simulink model "Earth_sim"  (R2024b)
settings: Solver=VariableStepAuto  StartTime=0.0  StopTime=15e4  FixedStep=0.5  MaxStep=10  RelTol=1e-6
undefined symbols (not defined in the file): earth_escape_data, Earth_planet, launch_data, launch_site, transfer_outbound_data
settings Model: Creator=cpero  LastModifiedBy=cpero
settings SolverCC: MaxConsecutiveMinStep=10  MinimalZcImpactIntegration=on  EnableFixedStepZeroCrossing=on
settings DebuggingCC: ReadBeforeWriteMsg=DisableAll  WriteAfterWriteMsg=DisableAll  WriteAfterReadMsg=DisableAll  MultiTaskDSMMsg=none
settings ModelReferenceCC: UpdateModelReferenceTargets=IfOutOfDate
settings SFSimCC: SFSimEcho=off

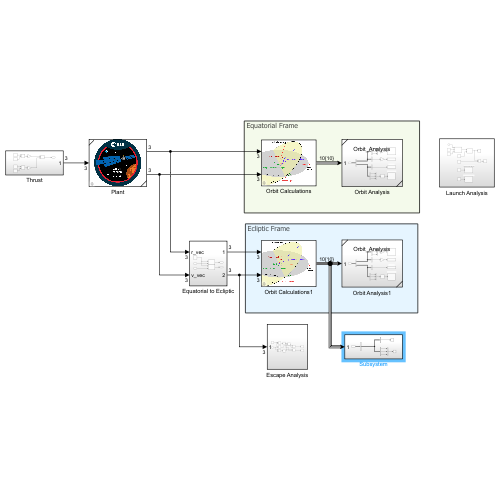
[thumbnail: Simulink's stored preview of the top-level diagram]
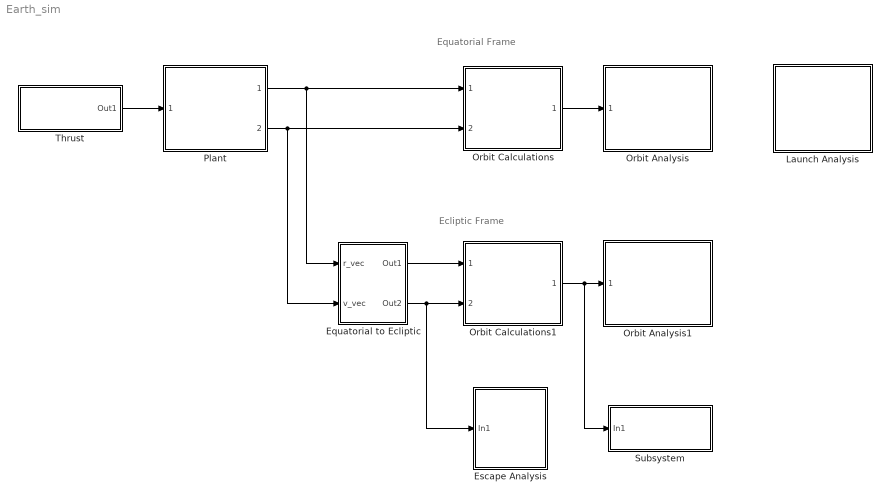
== system Earth_sim ==
  note: Equatorial Frame
  note: Ecliptic Frame
  Equatorial to Ecliptic : Subsystem
  Escape Analysis : Subsystem
  Launch Analysis : Subsystem
  Orbit Analysis : Subsystem  ReferencedSubsystem=Orbit_Analysis
  Orbit Analysis1 : Subsystem  ReferencedSubsystem=Orbit_Analysis
  Orbit Calculations : Subsystem  ReferencedSubsystem=Orbit_Calculations  mu=Earth_planet.mu
  Orbit Calculations1 : Subsystem  ReferencedSubsystem=Orbit_Calculations  mu=Earth_planet.mu
  Plant : Subsystem  ReferencedSubsystem=Plant  setup=launch_data  switch_time=launch_data.wait_time  mu=Earth_planet.mu
  Subsystem : Subsystem
  Thrust : Subsystem
  wires:
  Orbit Calculations/1 -> Orbit Analysis/1
  Plant/1 -> Orbit Calculations/1, Equatorial to Ecliptic/1(r_vec)
  Plant/2 -> Orbit Calculations/2, Equatorial to Ecliptic/2(v_vec)
  Orbit Calculations1/1 -> Subsystem/1(In1), Orbit Analysis1/1
  Equatorial to Ecliptic/1(Out1) -> Orbit Calculations1/1
  Equatorial to Ecliptic/2(Out2) -> Escape Analysis/1(In1), Orbit Calculations1/2
  Thrust/1(Out1) -> Plant/1

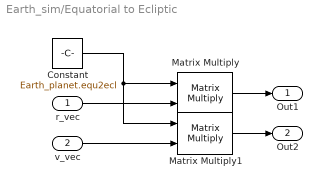
== system Earth_sim/Equatorial to Ecliptic ==
  r_vec : Inport
  v_vec : Inport  Port=2
  Constant : Constant  Value=Earth_planet.equ2ecl
  Matrix Multiply : Product  Multiplication=Matrix(*)
  Matrix Multiply1 : Product  Multiplication=Matrix(*)
  Out1 : Outport
  Out2 : Outport  Port=2
  wires:
  Constant/1 -> Matrix Multiply1/1, Matrix Multiply/1
  Matrix Multiply1/1 -> Out2/1
  Matrix Multiply/1 -> Out1/1
  r_vec/1 -> Matrix Multiply/2
  v_vec/1 -> Matrix Multiply1/2

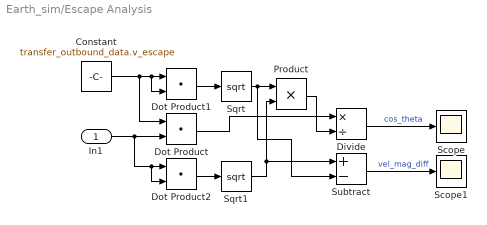
== system Earth_sim/Escape Analysis ==
  In1 : Inport
  Constant : Constant  Value=transfer_outbound_data.v_escape
  Divide : Product  Inputs=*/
  Dot Product : DotProduct  OutDataTypeStr=Inherit: Inherit via internal rule
  Dot Product1 : DotProduct  OutDataTypeStr=Inherit: Inherit via internal rule
  Dot Product2 : DotProduct  OutDataTypeStr=Inherit: Inherit via internal rule
  Product : Product
  Scope : Scope
  Scope1 : Scope
  Sqrt : Sqrt
  Sqrt1 : Sqrt
  Subtract : Sum  Inputs=+-
  wires:
  Constant/1 -> Dot Product1/2, Dot Product1/1, Dot Product/1
  Dot Product1/1 -> Sqrt/1
  Dot Product2/1 -> Sqrt1/1
  In1/1 -> Dot Product2/2, Dot Product2/1, Dot Product/2
  Sqrt/1 -> Subtract/2, Product/1
  Sqrt1/1 -> Product/2, Subtract/1
  Divide/1 -> Scope/1  "cos_theta"
  Product/1 -> Divide/2
  Dot Product/1 -> Divide/1
  Subtract/1 -> Scope1/1  "vel_mag_diff"

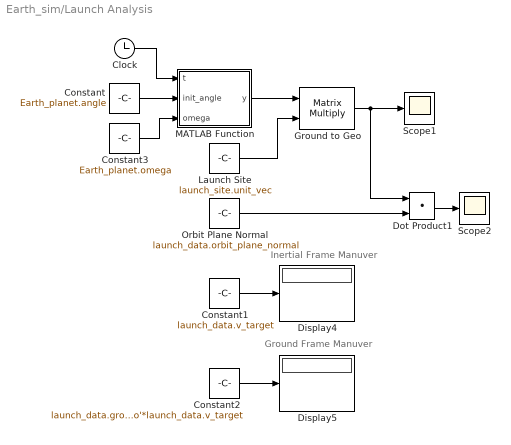
== system Earth_sim/Launch Analysis ==
  note: Ground Frame Manuver
  note: Inertial Frame Manuver
  Clock : Clock
  Constant : Constant  Value=Earth_planet.angle
  Constant1 : Constant  Value=launch_data.v_target
  Constant2 : Constant  Value=launch_data.ground2geo'*launch_data.v_target
  Constant3 : Constant  Value=Earth_planet.omega
  Display4 : Display
  Display5 : Display
  Dot Product1 : DotProduct  OutDataTypeStr=Inherit: Inherit via internal rule
  Ground to Geo : Product  Multiplication=Matrix(*)
  Launch Site : Constant  Value=launch_site.unit_vec
  MATLAB Function : MATLAB Function  TreatAsAtomicUnit=on
  Orbit Plane Normal : Constant  Value=launch_data.orbit_plane_normal
  Scope1 : Scope
  Scope2 : Scope
  wires:
  Dot Product1/1 -> Scope2/1
  Orbit Plane Normal/1 -> Dot Product1/2
  Ground to Geo/1 -> Scope1/1, Dot Product1/1
  Clock/1 -> MATLAB Function/1(t)
  MATLAB Function/1(y) -> Ground to Geo/1
  Launch Site/1 -> Ground to Geo/2
  Constant2/1 -> Display5/1
  Constant1/1 -> Display4/1
  Constant/1 -> MATLAB Function/2(init_angle)
  Constant3/1 -> MATLAB Function/3(omega)

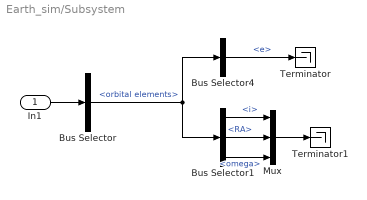
== system Earth_sim/Subsystem ==
  In1 : Inport
  Bus Selector : BusSelector  OutputSignals=orbital elements
  Bus Selector1 : BusSelector  OutputSignals=i,RA,omega
  Bus Selector4 : BusSelector  OutputSignals=e
  Mux : Mux  Inputs=3
  Terminator : Terminator
  Terminator1 : Terminator
  wires:
  Bus Selector1/3 -> Mux/3  "<omega>"
  Bus Selector4/1 -> Terminator/1  "<e>"
  Bus Selector1/2 -> Mux/2  "<RA>"
  Bus Selector/1 -> Bus Selector1/1, Bus Selector4/1  "<orbital elements>"
  Mux/1 -> Terminator1/1
  In1/1 -> Bus Selector/1
  Bus Selector1/1 -> Mux/1  "<i>"

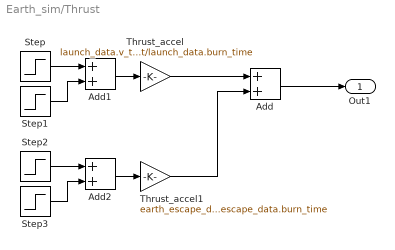
== system Earth_sim/Thrust ==
  Add : Sum
  Add1 : Sum
  Add2 : Sum
  Step : Step  Time=launch_data.wait_time  SampleTime=0
  Step1 : Step  Time=launch_data.wait_time + launch_data.burn_time  After=-1  SampleTime=0
  Step2 : Step  Time=launch_data.wait_time + earth_escape_data.time  SampleTime=0
  Step3 : Step  Time=launch_data.wait_time + earth_escape_data.time + earth_escape_data.burn_time  After=-1  SampleTime=0
  Thrust_accel : Gain  Gain=launch_data.v_target/launch_data.burn_time
  Thrust_accel1 : Gain  Gain=earth_escape_data.v_target/earth_escape_data.burn_time
  Out1 : Outport
  wires:
  Add1/1 -> Thrust_accel/1
  Step2/1 -> Add2/1
  Step1/1 -> Add1/2
  Add2/1 -> Thrust_accel1/1
  Step3/1 -> Add2/2
  Step/1 -> Add1/1
  Thrust_accel/1 -> Add/1
  Thrust_accel1/1 -> Add/2
  Add/1 -> Out1/1

== matlab function Earth_sim/Launch Analysis/MATLAB Function ==
  data: y output; t input; init_angle input; omega input
function y = fcn(t, init_angle, omega)

y = [cos(omega*t + init_angle), -sin(omega*t + init_angle), 0;
     sin(omega*t + init_angle), cos(omega*t + init_angle), 0;
     0, 0, 1];
